simulink model "labkit1test"  (R2021a)
settings: Solver=FixedStepDiscrete  StartTime=0.0  StopTime=inf  RelTol=1e-3  EnableMultiTasking=on
libraries: labkit_toolbox x5, canmsglib x2
settings Model: Creator=user  LastModifiedBy=madhe
settings SolverCC: PositivePriorityOrder=on  AutoInsertRateTranBlk=on
settings OptimizationCC: DefaultParameterBehavior=Inlined  EnhancedBackFolding=on  PassReuseOutputArgsAs=Individual arguments  ZeroExternalMemoryAtStartup=off  ZeroInternalMemoryAtStartup=off  OptimizeBlockOrder=speed  DifferentSizesBufferReuse=on  OptimizationCustomize=off  EfficientTunableParamExpr=on
settings DebuggingCC: ParameterTunabilityLossMsg=error
settings SFSimCC: MATLABDynamicMemAlloc=off
settings RTWCC: Description=Waijung 2 ESP32 target  SystemTargetFile=esp32.tlc  GenCodeOnly=on  MakeCommand=make_rtw TMF=1  GenerateMakefile=off  TemplateMakefile=ert_default_tmf  RetainRTWFile=on
settings CodeAppCC: ForceParamTrailComments=on  IgnoreCustomStorageClasses=off  OperatorAnnotations=on  SimulinkDataObjDesc=on  SFDataObjDesc=on  InsertBlockDesc=on
settings ERTTargetCC: TargetLangStandard=C99 (ISO)  UseToolchainInfoCompliant=off  InlinedParameterPlacement=NonHierarchical  ERTSrcFileBannerTemplate=esp32_code_template.cgt  ERTHdrFileBannerTemplate=esp32_code_template.cgt  ERTDataSrcFileTemplate=esp32_code_template.cgt  ERTDataHdrFileTemplate=esp32_code_template.cgt  ERTCustomFileTemplate=esp32_file_process.tlc

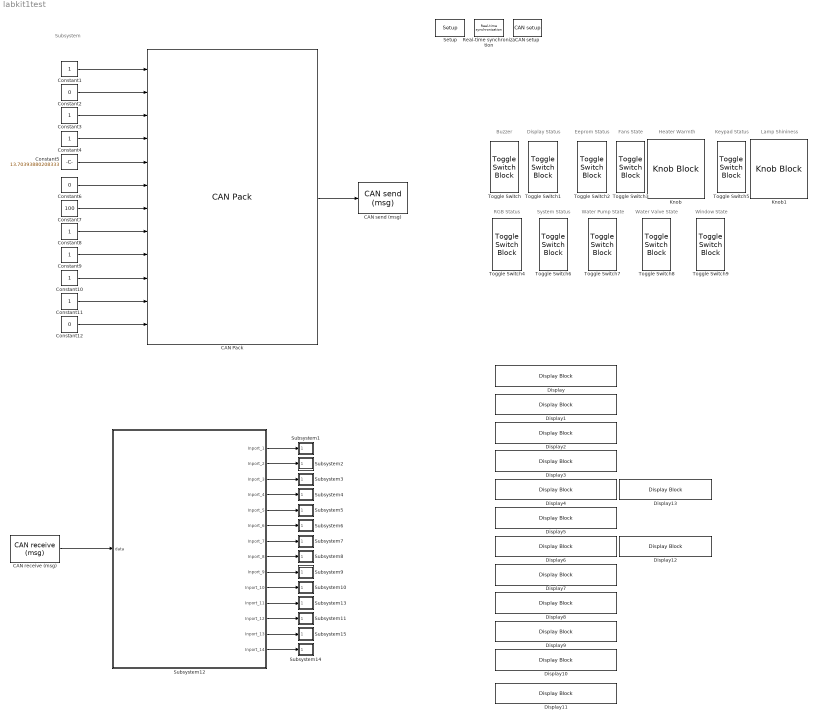
== system labkit1test ==
  note: Subsystem
  note: Window State
  note: Water Valve State
  note: Water Pump State
  note: System Status
  note: RGB Status
  note: Lamp Shininess
  note: Keypad Status
  note: Heater Warmth
  note: Fans State
  note: Eeprom Status
  note: Display Status
  note: Buzzer
  CAN Pack : canmsglib/CAN Pack  CANdbFile=C:\Users\user\Documents\SoftwareTesterStuff\Greenhouse Stuff\greenhouse.dbc  MsgList=(none)  MsgName=hmi  MsgIDType=Standard (11-bit identifier)  MsgIdentifier=258  MsgLength=8  Remote=off  ApplyMinMax=off  BusOutput=on  SignalInfo={'buzzer_status','40','2','LE','unsigned','Standard','0','1','0','-Inf','Inf';'display_status','36','2','LE','unsigned','Standard','0','1','0','-Inf','Inf';'eeprom_status','44','2','LE','unsigned','Standard','0','1','0','-Inf','Inf';'fans_state','22','1','LE','unsigned','Standard','0','1','0','-Inf','Inf';'heater_warmness','8','7','LE','unsigned','Standard','0','1','0','0','100';'keypad_status','38','2','LE','unsigned','Standard','0','1','0','-Inf','Inf';'lamp_shininess','0','7','LE','unsigned','Standard','0','1','0','0','100';'rgb_status','42','2','LE','unsigned','Standard','0','1','0','-Inf','Inf';'system_status','46','2','LE','unsigned','Standard','0','1','0','-Inf','Inf';'water_pump_state','16','1','LE','unsigned','Standard','0','1','0','-Inf','Inf';'water_valve_state','18','1','LE','unsigned','Standard','0','1','0','-Inf','Inf';'window_state','20','1','LE','unsigned','Standard','0','1','0','-Inf','Inf'}
      settings: SourceProductBaseCode=ME,XP,VN  DataFormat=CANdb specified signals
  CAN receive (msg) : labkit_toolbox/CAN receive (msg)  frame_id=258  sample_time=0.5
      settings: SourceProductName=Lab kit toolbox
  CAN send (msg) : labkit_toolbox/CAN send (msg)  frame_id=0x102  sample_time=0.5
      settings: SourceProductName=Lab kit toolbox
  CAN setup : labkit_toolbox/CAN setup  brp=10  tseg1=8  tseg2=7  sjw=1
      settings: SourceProductName=Lab kit toolbox
  Constant1 : Constant  VectorParams1D=off  OutDataTypeStr=uint8  SampleTime=0.1
  Constant{3..4,8..11} (6 alike) : Constant
  Constant12 : Constant  Value=0
  Constant2 : Constant  Value=0
  Constant5 : Constant  Value=13.70393880208333
  Constant6 : Constant  Value=0
  Constant7 : Constant  Value=100
  Display{,1..13} (14 alike) : DisplayBlock  LabelPosition=Hide  Format=short  Transparency=1
  Knob : KnobBlock
  Knob1 : KnobBlock
  Real-time synchronization : labkit_toolbox/Real-time synchronization  time_step=0.1
      settings: SourceProductName=Lab kit toolbox
  Setup : labkit_toolbox/Setup  port=COM3
      settings: SourceProductName=Lab kit toolbox
  Subsystem1 : Subsystem
  Subsystem10 : Subsystem
  Subsystem11 : Subsystem
  Subsystem12 : Subsystem
  Subsystem13 : Subsystem
  Subsystem14 : Subsystem
  Subsystem15 : Subsystem
  Subsystem2 : Subsystem
  Subsystem3 : Subsystem
  Subsystem4 : Subsystem
  Subsystem5 : Subsystem
  Subsystem6 : Subsystem
  Subsystem7 : Subsystem
  Subsystem8 : Subsystem
  Subsystem9 : Subsystem
  Toggle Switch{,1..9} (10 alike) : ToggleSwitchBlock
      settings: Values={{'Off', 'On'}, [0 1]}
  wires:
  CAN receive (msg)/1 -> Subsystem12/1(data)
  CAN Pack/1 -> CAN send (msg)/1
  Subsystem12/1(Inport_1) -> Subsystem1/1(In1)
  Subsystem12/2(Inport_2) -> Subsystem2/1(Inport_2)
  Subsystem12/3(Inport_3) -> Subsystem3/1(In1)
  Subsystem12/4(Inport_4) -> Subsystem4/1(Inport_2)
  Subsystem12/5(Inport_5) -> Subsystem5/1(In1)
  Subsystem12/6(Inport_6) -> Subsystem6/1(Inport_2)
  Subsystem12/7(Inport_7) -> Subsystem7/1(In1)
  Subsystem12/8(Inport_8) -> Subsystem8/1(Inport_2)
  Subsystem12/9(Inport_9) -> Subsystem9/1(In1)
  Subsystem12/10(Inport_10) -> Subsystem10/1(Inport_2)
  Subsystem12/11(Inport_11) -> Subsystem13/1(Inport_11)
  Subsystem12/12(Inport_12) -> Subsystem11/1(Inport_2)
  Subsystem12/13(Inport_13) -> Subsystem15/1(Inport_13)
  Subsystem12/14(Inport_14) -> Subsystem14/1(Inport_2)
  Constant5/1 -> CAN Pack/5
  Constant11/1 -> CAN Pack/11
  Constant8/1 -> CAN Pack/8
  Constant9/1 -> CAN Pack/9
  Constant12/1 -> CAN Pack/12
  Constant10/1 -> CAN Pack/10
  Constant6/1 -> CAN Pack/6
  Constant3/1 -> CAN Pack/3
  Constant2/1 -> CAN Pack/2
  Constant1/1 -> CAN Pack/1
  Constant4/1 -> CAN Pack/4
  Constant7/1 -> CAN Pack/7

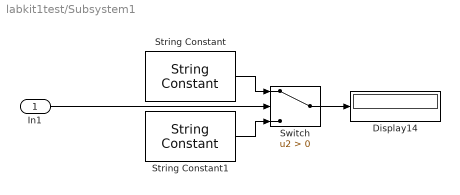
== system labkit1test/Subsystem1 ==
  In1 : Inport
  Display14 : Display
  String Constant : StringConstant  String="\"Buzzer is ON\""
  String Constant1 : StringConstant  String="\"Buzzer is OFF\""
  Switch : Switch  Criteria=u2 > Threshold
  wires:
  In1/1 -> Switch/2
  String Constant1/1 -> Switch/3
  Switch/1 -> Display14/1
  String Constant/1 -> Switch/1

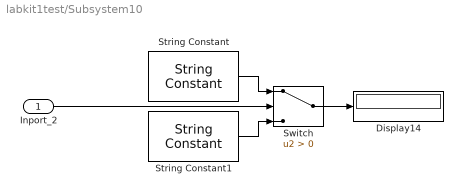
== system labkit1test/Subsystem10 ==
  Inport_2 : Inport
  Display14 : Display
  String Constant : StringConstant  String="\"RGB is ON\""
  String Constant1 : StringConstant  String="\"RGB is OFF\""
  Switch : Switch  Criteria=u2 > Threshold
  wires:
  Inport_2/1 -> Switch/2
  String Constant1/1 -> Switch/3
  Switch/1 -> Display14/1
  String Constant/1 -> Switch/1

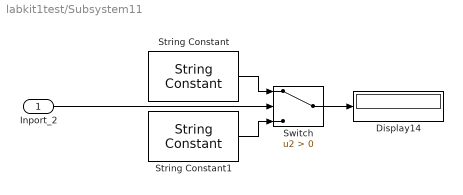
== system labkit1test/Subsystem11 ==
  Inport_2 : Inport
  Display14 : Display
  String Constant : StringConstant  String="\"Water Pump is ON\""
  String Constant1 : StringConstant  String="\"Water Pump is OFF\""
  Switch : Switch  Criteria=u2 > Threshold
  wires:
  Inport_2/1 -> Switch/2
  String Constant1/1 -> Switch/3
  Switch/1 -> Display14/1
  String Constant/1 -> Switch/1

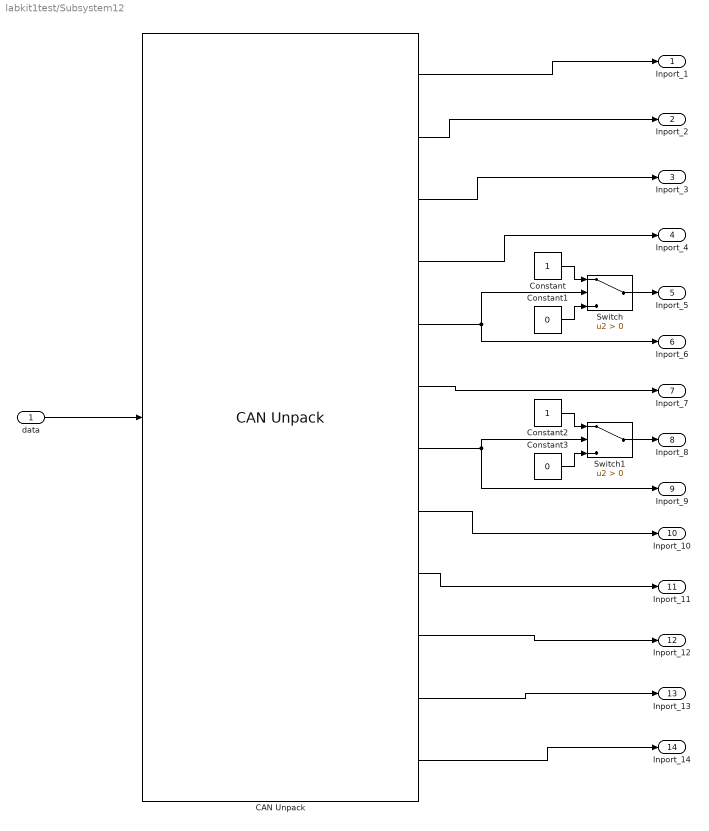
== system labkit1test/Subsystem12 ==
  data : Inport
  CAN Unpack : canmsglib/CAN Unpack  CANdbFile=C:\Users\user\Documents\SoftwareTesterStuff\Greenhouse Stuff\greenhouse.dbc  MsgList=(none)  MsgName=hmi  MsgIDType=Standard (11-bit identifier)  MsgIdentifier=258  MsgLength=8  SignalInfo={'buzzer_status','40','2','LE','unsigned','Standard','0','1','0','-Inf','Inf';'display_status','36','2','LE','unsigned','Standard','0','1','0','-Inf','Inf';'eeprom_status','44','2','LE','unsigned','Standard','0','1','0','-Inf','Inf';'fans_state','22','1','LE','unsigned','Standard','0','1','0','-Inf','Inf';'heater_warmness','8','7','LE','unsigned','Standard','0','1','0','0','100';'keypad_status','38','2','LE','unsigned','Standard','0','1','0','-Inf','Inf';'lamp_shininess','0','7','LE','unsigned','Standard','0','1','0','0','100';'rgb_status','42','2','LE','unsigned','Standard','0','1','0','-Inf','Inf';'system_status','46','2','LE','unsigned','Standard','0','1','0','-Inf','Inf';'water_pump_state','16','1','LE','unsigned','Standard','0','1','0','-Inf','Inf';'water_valve_state','18','1','LE','unsigned','Standard','0','1','0','-Inf','Inf';'window_state','20','1','LE','unsigned','Standard','0','1','0','-Inf','Inf'}  IDPort=off  TimestampPort=off  ErrorPort=off  RemotePort=off  LengthPort=off  StatusPort=off  ApplyMinMax=off
      settings: SourceProductBaseCode=ME,XP,VN  DataFormat=CANdb specified signals
  Constant : Constant
  Constant1 : Constant  Value=0
  Constant2 : Constant
  Constant3 : Constant  Value=0
  Switch : Switch  Criteria=u2 > Threshold
  Switch1 : Switch  Criteria=u2 > Threshold
  Inport_1 : Outport
  Inport_2 : Outport  Port=2
  Inport_3 : Outport  Port=3
  Inport_4 : Outport  Port=4
  Inport_5 : Outport  Port=5
  Inport_6 : Outport  Port=6
  Inport_7 : Outport  Port=7
  Inport_8 : Outport  Port=8
  Inport_9 : Outport  Port=9
  Inport_10 : Outport  Port=10
  Inport_11 : Outport  Port=11
  Inport_12 : Outport  Port=12
  Inport_13 : Outport  Port=13
  Inport_14 : Outport  Port=14
  wires:
  CAN Unpack/1 -> Inport_1/1
  Switch1/1 -> Inport_8/1
  Constant3/1 -> Switch1/3
  Constant2/1 -> Switch1/1
  CAN Unpack/7 -> Inport_9/1, Switch1/2
  Switch/1 -> Inport_5/1
  Constant/1 -> Switch/1
  Constant1/1 -> Switch/3
  CAN Unpack/6 -> Inport_7/1
  CAN Unpack/3 -> Inport_3/1
  CAN Unpack/12 -> Inport_14/1
  CAN Unpack/2 -> Inport_2/1
  CAN Unpack/4 -> Inport_4/1
  CAN Unpack/11 -> Inport_13/1
  CAN Unpack/8 -> Inport_10/1
  CAN Unpack/10 -> Inport_12/1
  CAN Unpack/5 -> Inport_6/1, Switch/2
  CAN Unpack/9 -> Inport_11/1
  data/1 -> CAN Unpack/1

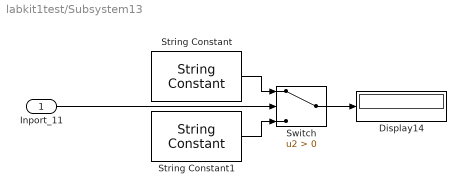
== system labkit1test/Subsystem13 ==
  Inport_11 : Inport
  Display14 : Display
  String Constant : StringConstant  String="\"System is ON\""
  String Constant1 : StringConstant  String="\"System is OFF\""
  Switch : Switch  Criteria=u2 > Threshold
  wires:
  Inport_11/1 -> Switch/2
  String Constant1/1 -> Switch/3
  Switch/1 -> Display14/1
  String Constant/1 -> Switch/1

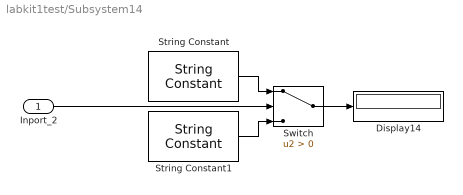
== system labkit1test/Subsystem14 ==
  Inport_2 : Inport
  Display14 : Display
  String Constant : StringConstant  String="\"Window is ON\""
  String Constant1 : StringConstant  String="\"Window is OFF\""
  Switch : Switch  Criteria=u2 > Threshold
  wires:
  Inport_2/1 -> Switch/2
  String Constant1/1 -> Switch/3
  Switch/1 -> Display14/1
  String Constant/1 -> Switch/1

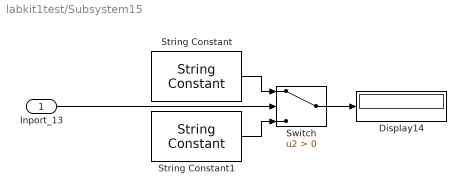
== system labkit1test/Subsystem15 ==
  Inport_13 : Inport
  Display14 : Display
  String Constant : StringConstant  String="\"Water Valve is ON\""
  String Constant1 : StringConstant  String="\"Water Valve is OFF\""
  Switch : Switch  Criteria=u2 > Threshold
  wires:
  Inport_13/1 -> Switch/2
  String Constant1/1 -> Switch/3
  Switch/1 -> Display14/1
  String Constant/1 -> Switch/1

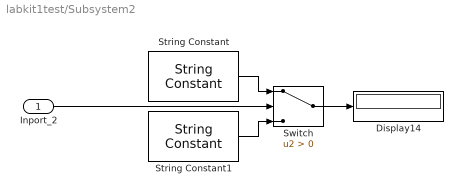
== system labkit1test/Subsystem2 ==
  Inport_2 : Inport
  Display14 : Display
  String Constant : StringConstant  String="\"Display is ON\""
  String Constant1 : StringConstant  String="\"Display is OFF\""
  Switch : Switch  Criteria=u2 > Threshold
  wires:
  Inport_2/1 -> Switch/2
  String Constant1/1 -> Switch/3
  Switch/1 -> Display14/1
  String Constant/1 -> Switch/1

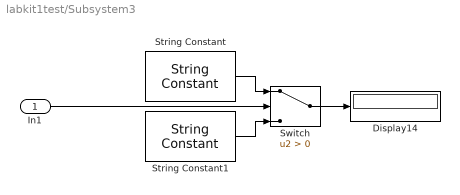
== system labkit1test/Subsystem3 ==
  In1 : Inport
  Display14 : Display
  String Constant : StringConstant  String="\"EEprom is ON\""
  String Constant1 : StringConstant  String="\"EEprom is OFF\""
  Switch : Switch  Criteria=u2 > Threshold
  wires:
  In1/1 -> Switch/2
  String Constant1/1 -> Switch/3
  Switch/1 -> Display14/1
  String Constant/1 -> Switch/1

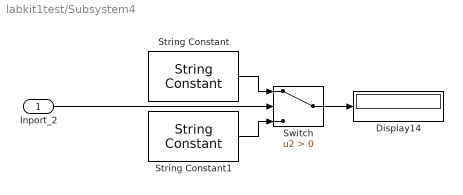
== system labkit1test/Subsystem4 ==
  Inport_2 : Inport
  Display14 : Display
  String Constant : StringConstant  String="\"Fans are ON\""
  String Constant1 : StringConstant  String="\"Fans are OFF\""
  Switch : Switch  Criteria=u2 > Threshold
  wires:
  Inport_2/1 -> Switch/2
  String Constant1/1 -> Switch/3
  Switch/1 -> Display14/1
  String Constant/1 -> Switch/1

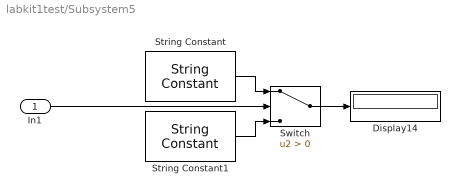
== system labkit1test/Subsystem5 ==
  In1 : Inport
  Display14 : Display
  String Constant : StringConstant  String="\"Heater is ON and its value is\""
  String Constant1 : StringConstant  String="\"Buzzer is OFF\""
  Switch : Switch  Criteria=u2 > Threshold
  wires:
  In1/1 -> Switch/2
  String Constant1/1 -> Switch/3
  Switch/1 -> Display14/1
  String Constant/1 -> Switch/1

== system labkit1test/Subsystem6 ==
  Inport_2 : Inport
  Display14 : Display
  String Constant : StringConstant  String="\"Display is ON\""
  String Constant1 : StringConstant  String="\"Display is OFF\""
  Switch : Switch  Criteria=u2 > Threshold
  wires:
  Inport_2/1 -> Switch/2
  String Constant1/1 -> Switch/3
  Switch/1 -> Display14/1
  String Constant/1 -> Switch/1

== system labkit1test/Subsystem7 ==
  In1 : Inport
  Display14 : Display
  String Constant : StringConstant  String="\"Keypad is ON\""
  String Constant1 : StringConstant  String="\"Keypad is OFF\""
  Switch : Switch  Criteria=u2 > Threshold
  wires:
  In1/1 -> Switch/2
  String Constant1/1 -> Switch/3
  Switch/1 -> Display14/1
  String Constant/1 -> Switch/1

== system labkit1test/Subsystem8 ==
  Inport_2 : Inport
  Display14 : Display
  String Constant : StringConstant  String="\"Lamp is ON and its value is\""
  String Constant1 : StringConstant  String="\"Lamp is OFF\""
  Switch : Switch  Criteria=u2 > Threshold
  wires:
  Inport_2/1 -> Switch/2
  String Constant1/1 -> Switch/3
  Switch/1 -> Display14/1
  String Constant/1 -> Switch/1

== system labkit1test/Subsystem9 ==
  In1 : Inport
  Display14 : Display
  String Constant : StringConstant  String="\"Buzzer is ON\""
  String Constant1 : StringConstant  String="\"Buzzer is OFF\""
  Switch : Switch  Criteria=u2 > Threshold
  wires:
  In1/1 -> Switch/2
  String Constant1/1 -> Switch/3
  Switch/1 -> Display14/1
  String Constant/1 -> Switch/1
